simulink model "Variable_mass_matrix_harness"  (R2020b)
settings: Solver=ode4  StartTime=0.0  StopTime=par.sym.Ttot  FixedStep=0.05  MaxStep=par.sym.max_dt  RelTol=1e-3
settings Model: Creator=carar  LastModifiedBy=carar
settings SolverCC: AlgebraicLoopSolver=LineSearch
settings DataIOCC: SaveOutput=off  SaveTime=off  ReturnWorkspaceOutputs=off  TimeSaveName=TIME
settings OptimizationCC: LifeSpan=inf
settings DebuggingCC: UnconnectedInputMsg=none  UnconnectedOutputMsg=none  ArithmeticOperatorsInVariantConditions=warning
settings SFSimCC: CustomCodeUndefinedFunction=UseInterfaceOnly
settings CodeAppCC: GenerateComments=off
settings SimscapeCC: SimscapeNormalizeSystem=off

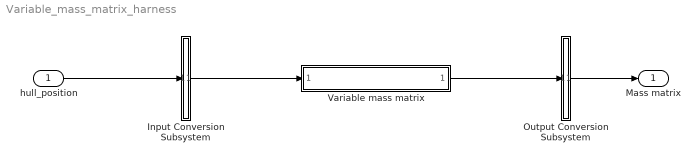
== system Variable_mass_matrix_harness ==
  hull_position : Inport  OutDataTypeStr=double  PortDimensions=[6]  SampleTime=0.05
  Input Conversion Subsystem : Subsystem  Tag=__SLT_ICS__  Description=|
      | Signal spec.
      | and routing
      settings: AttributesFormatString=%<Description>
  Output Conversion Subsystem : Subsystem  Tag=__SLT_OCS__  Description=|
      | Signal spec.
      | and routing
      settings: AttributesFormatString=%<Description>
  Variable mass matrix : ModelReference  ModelNameDialog=Variable_mass_matrix.slxp  ModelReferenceVersion=5.19  CopyOfModelProtected=on
  Mass matrix : Outport
  wires:
  hull_position/1 -> Input Conversion Subsystem/1(Inport_1)
  Output Conversion Subsystem/1(Outport_1) -> Mass matrix/1
  Input Conversion Subsystem/1(Outport_1) -> Variable mass matrix/1
  Variable mass matrix/1 -> Output Conversion Subsystem/1(Inport_1)

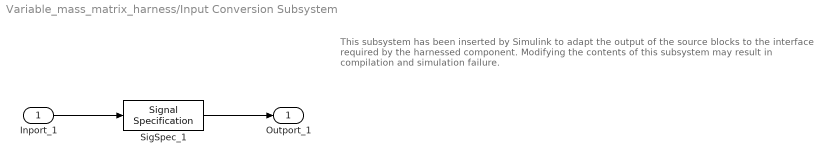
== system Variable_mass_matrix_harness/Input Conversion Subsystem ==
  note: This subsystem has been inserted by Simulink to adapt the output of the source blocks to the interface required by the harnessed component.
      |  Modifying the contents of this subsystem may result in compilation and simulation failure.
  Inport_1 : Inport
  SigSpec_1 : SignalSpecification  OutDataTypeStr=double  Dimensions=[6]  SampleTime=0.05
  Outport_1 : Outport
  wires:
  SigSpec_1/1 -> Outport_1/1
  Inport_1/1 -> SigSpec_1/1

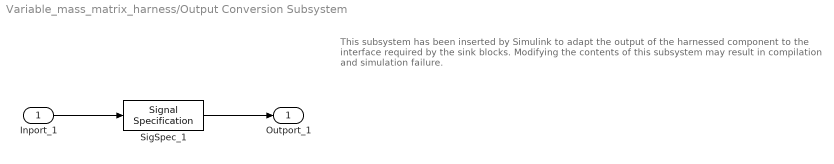
== system Variable_mass_matrix_harness/Output Conversion Subsystem ==
  note: This subsystem has been inserted by Simulink to adapt the output of the harnessed component to the interface required by the sink blocks.
      |  Modifying the contents of this subsystem may result in compilation and simulation failure.
  Inport_1 : Inport
  SigSpec_1 : SignalSpecification  OutDataTypeStr=double  Dimensions=[6, 6]  SampleTime=0.05
  Outport_1 : Outport
  wires:
  Inport_1/1 -> SigSpec_1/1
  SigSpec_1/1 -> Outport_1/1
